simulink model "Maglev_NMPC_AcadosSim"  (R2025a)
settings: Solver=ode23t  StartTime=0.0  StopTime=T_sim  FixedStep=mpc.Ts  MaxStep=0.0001  RelTol=1e-4
PreLoadFcn:
  | modelPath = fileparts(which(bdroot));
  | projectRoot = fileparts(modelPath);
  | 
  | run(fullfile(projectRoot, 'setup_sim_params.m'));
  | load(fullfile(projectRoot, 'Controller_Params', 'StandardNMPCData.mat'));
  | % Add the generated code folder so Simulink can find the mexw64
  | addpath(fullfile(projectRoot, 'Controller_Design/design_nmpc/c_generated_code'))
  | addpath(fullfile(projectRoot, 'Controller_Design/design_nmpc/c_generated_code/singleMaglev_model'))
  | 
  | load('sfun_port_names')
undefined symbols (not defined in the file): airgap_eq, nmpc
settings Model: Creator=Polarstern  LastModifiedBy=CelestialAurora

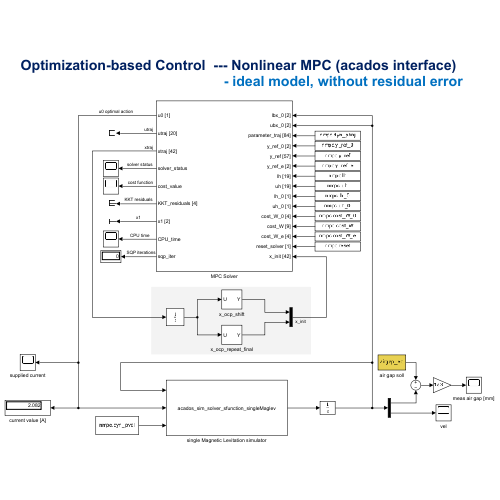
[thumbnail: Simulink's stored preview of the top-level diagram]
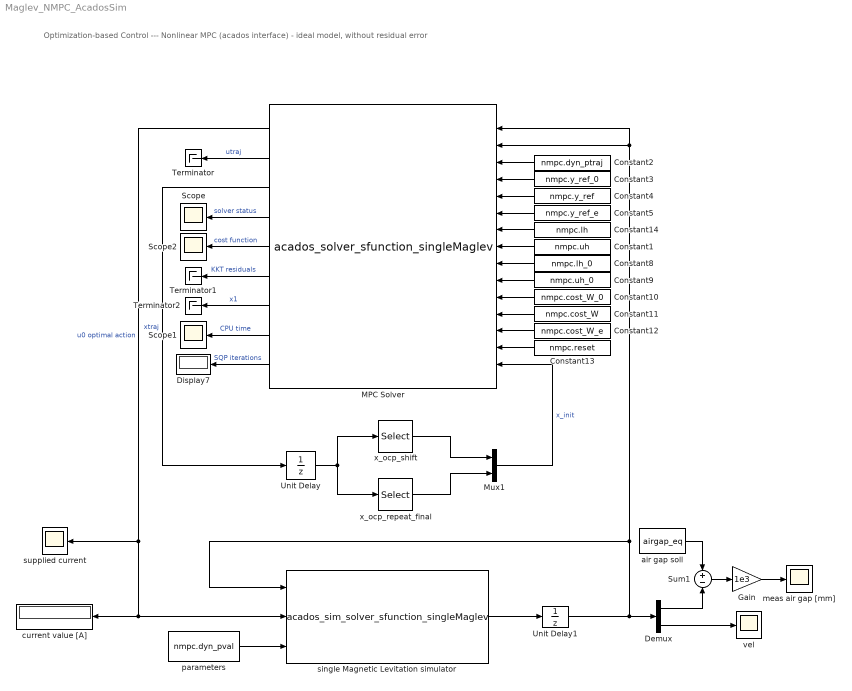
== system Maglev_NMPC_AcadosSim ==
  note: Optimization-based Control --- Nonlinear MPC (acados interface)
      | - ideal model, without residual error
  Constant1 : Constant  Value=nmpc.uh
  Constant10 : Constant  Value=nmpc.cost_W_0
  Constant11 : Constant  Value=nmpc.cost_W
  Constant12 : Constant  Value=nmpc.cost_W_e
  Constant13 : Constant  Value=nmpc.reset
  Constant14 : Constant  Value=nmpc.lh
  Constant2 : Constant  Value=nmpc.dyn_ptraj
  Constant3 : Constant  Value=nmpc.y_ref_0
  Constant4 : Constant  Value=nmpc.y_ref
  Constant5 : Constant  Value=nmpc.y_ref_e
  Constant8 : Constant  Value=nmpc.lh_0
  Constant9 : Constant  Value=nmpc.uh_0
  Demux : Demux  Outputs=2
  Display7 : Display
  Gain : Gain  Gain=1e3
  MPC Solver : S-Function  FunctionName=acados_solver_sfunction_singleMaglev  SFunctionDeploymentMode=off  EnableBusSupport=off
      mask Display:
      | global sfun_input_names sfun_output_names
      | for i = 1:length(sfun_input_names)
      | 	port_label('input', i, sfun_input_names{i})
      | end
      | for i = 1:length(sfun_output_names)
      | 	port_label('output', i, sfun_output_names{i})
      | end
  Mux1 : Mux  Inputs=2
  Scope : Scope
      settings: ActiveDisplayYMinimum=-1  ActiveDisplayYMaximum=1
  Scope1 : Scope
      settings: ActiveDisplayYMinimum=-0.00038942499999999988  ActiveDisplayYMaximum=0.0041428249999999993  DataLoggingVariableName=ScopeData2
  Scope2 : Scope
      settings: ActiveDisplayYMinimum=-1  ActiveDisplayYMaximum=1  DataLoggingVariableName=ScopeData4
  Sum1 : Sum  Inputs=+|-
  Terminator : Terminator
  Terminator1 : Terminator
  Terminator2 : Terminator
  Unit Delay : UnitDelay  InitialCondition=nmpc.x_init  SampleTime=nmpc.Ts  HasFrameUpgradeWarning=on
  Unit Delay1 : UnitDelay  InitialCondition=nmpc.x_init_con  SampleTime=0.0001  HasFrameUpgradeWarning=on
  air gap soll : Constant  Value=airgap_eq
  current value [A] : Display
  meas air gap [mm] : Scope
      settings: ActiveDisplayYMinimum=1.9374847718520893  ActiveDisplayYMaximum=2.5625016920164345  DataLoggingVariableName=ScopeData5
  parameters : Constant  Value=nmpc.dyn_pval
  single Magnetic Levitation simulator : S-Function  FunctionName=acados_sim_solver_sfunction_singleMaglev  SFunctionDeploymentMode=off  EnableBusSupport=off
  supplied current : Scope
      settings: ActiveDisplayYMinimum=-1  ActiveDisplayYMaximum=1  DataLoggingVariableName=ScopeData7
  vel : Scope
      settings: ActiveDisplayYMinimum=-0.0014909131187886091  ActiveDisplayYMaximum=0.013397000226356955  DataLoggingVariableName=ScopeData6
  x_ocp_repeat_final : Selector  IndexMode=Zero-based  InputPortWidth=(nmpc.N+1)*nmpc.nx  IndexOptions=Starting index (dialog)  Indices=nmpc.N*nmpc.nx  OutputSizes=nmpc.nx
  x_ocp_shift : Selector  IndexMode=Zero-based  InputPortWidth=(nmpc.N+1)*nmpc.nx  IndexOptions=Starting index (dialog)  Indices=nmpc.nx  OutputSizes=nmpc.N*nmpc.nx
  wires:
  MPC Solver/1 -> current value [A]/1, single Magnetic Levitation simulator/2, supplied current/1  "u0 optimal action"
  MPC Solver/2 -> Terminator/1  "utraj"
  MPC Solver/3 -> Unit Delay/1  "xtraj"
  MPC Solver/4 -> Scope/1  "solver status"
  MPC Solver/5 -> Scope2/1  "cost function"
  MPC Solver/6 -> Terminator1/1  "KKT residuals"
  MPC Solver/7 -> Terminator2/1  "x1"
  MPC Solver/8 -> Scope1/1  "CPU time"
  MPC Solver/9 -> Display7/1  "SQP iterations"
  Unit Delay/1 -> x_ocp_repeat_final/1, x_ocp_shift/1
  x_ocp_repeat_final/1 -> Mux1/2
  x_ocp_shift/1 -> Mux1/1
  single Magnetic Levitation simulator/1 -> Unit Delay1/1
  parameters/1 -> single Magnetic Levitation simulator/3
  Demux/2 -> vel/1
  Demux/1 -> Sum1/2
  air gap soll/1 -> Sum1/1
  Sum1/1 -> Gain/1
  Constant2/1 -> MPC Solver/3
  Constant3/1 -> MPC Solver/4
  Constant4/1 -> MPC Solver/5
  Constant5/1 -> MPC Solver/6
  Constant14/1 -> MPC Solver/7
  Constant1/1 -> MPC Solver/8
  Constant8/1 -> MPC Solver/9
  Constant9/1 -> MPC Solver/10
  Constant10/1 -> MPC Solver/11
  Constant11/1 -> MPC Solver/12
  Constant12/1 -> MPC Solver/13
  Constant13/1 -> MPC Solver/14
  Mux1/1 -> MPC Solver/15  "x_init"
  Unit Delay1/1 -> single Magnetic Levitation simulator/1, MPC Solver/1, MPC Solver/2, Demux/1
  Gain/1 -> meas air gap [mm]/1
